simulink model "P3_Ex12b"  (R2018a)
settings: Solver=FixedStepAuto  StartTime=0.0  StopTime=30  RelTol=1e-3
PreLoadFcn:
  | % Plant
  | K0=0.82/0.017;
  | tau0=0.26;
  | N=9;
  | Kpot=1.62;
  | % Sampling period
  | Ts=0.01;
  | 
  | % Desired control specifications
  | Sp=80; % overshoot
  | Fd=0.5; % frequency
  | 
  | % Poles of the second order continuous system that will fulfill the specifications
  | wd=2*pi*Fd ;
  | xi=sqrt((log(Sp/100))^2/(pi^2+log(Sp/100)^2))
  | wn=wd/ sqrt(1-xi^2)
  | s1=-xi*wn+j*wd
  | s2=-xi*wn-j*wd
  | 
  | % Poles of the second order discrete system that will fulfill the specifications
  | p1=exp(Ts* s1 )
  | p2=exp(Ts* s2 )
  | % Fix third pole
  | p3=0.01
  | 
  | % Plant's Z transfere function
  | Ptas=tf([K0*(1/N)*Kpot],[tau0,1,0]);
  | Ptaz=c2d(Ptas,Ts,'zoh');
  | 
  | % Denominator and numerator coefficients
  | [Nz ,Dz]= tfdata(Ptaz,'v')
  | a1=Nz(2);
  | a0=Nz(3);
  | b1=Dz(2);
  | b0=Dz(3);
  | 
  | % A and B matrix definitions
  | A=[-1 -a1 -a1 -a1 ; p2+p3+p1 a1-a0 -a1-a0 -a0+2*a1 ; ...
  |    -p1*p2-p3*p1-p2*p3 a0 -a0 2*a0-a1 ; p1*p2*p3 0 0 -a0 ] ;
  | b=[p1+p2+p3-1+b1 ; -p1*p2-p3*p1-p3*p2+b0-b1 ; p1*p2*p3-b0 ; 0 ] ;
  | 
  | % x vector's determination of the controller
  | x=inv(A)*b ;
  | 
  | p4=x(1)
  | Kp=x(2)
  | Ki=(2/Ts)*x(3)
  | Kd=Ts*x(4)
  | pawd=0.2;
  | Kaw=1/Ki;
  | 
  | % Poles dominance calculation
  | dominancia=log(abs(p4))/log(abs(p1))
undefined symbols (not defined in the file or in its folder): DiscIntNeverNeededParam
libraries: arduinolib x2, simulink x2
settings Model: SimulationMode=external  ExtModeTrigDuration=2  Creator=Eneko Lerma  LastModifiedBy=Eneko Lerma
settings OptimizationCC: EnhancedBackFolding=on  PassReuseOutputArgsAs=Individual arguments  MaxStackSize=64  OptimizeBlockOrder=speed  DifferentSizesBufferReuse=on  OptimizationCustomize=off
settings DebuggingCC: ParameterPrecisionLossMsg=none  ParameterTunabilityLossMsg=error
settings HardwareCC: ProdBitPerPointer=32  ProdBitPerSizeT=32  ProdBitPerPtrDiffT=32  ProdLargestAtomicInteger=Long  ProdLargestAtomicFloat=Double  ProdWordSize=32  ProdHWDeviceType=ARM Compatible->ARM Cortex
settings SFSimCC: MATLABDynamicMemAlloc=off
settings RTWCC: SystemTargetFile=ert.tlc  HardwareBoard=Arduino Due  TLCOptions=-aInlineSetEventsForThisBaseRateFcn=TLC_FALSE -aSuppressMultiTaskScheduler=TLC_FALSE -aRateBasedStepFcn=1  TemplateMakefile=ert_default_tmf  GenerateReport=on  Toolchain=Arduino ARM  BuildConfiguration=Faster Runs  IncludeHyperlinkInReport=on  LaunchReport=on  GenerateTraceInfo=on  GenerateTraceReport=on  GenerateTraceReportSl=on  GenerateTraceReportSf=on  GenerateTraceReportEml=on
settings CodeAppCC: ForceParamTrailComments=on  IgnoreCustomStorageClasses=off  OperatorAnnotations=on  SimulinkDataObjDesc=on  SFDataObjDesc=on  InsertBlockDesc=on
settings ERTTargetCC: SupportContinuousTime=on  SupportVariableSizeSignals=on

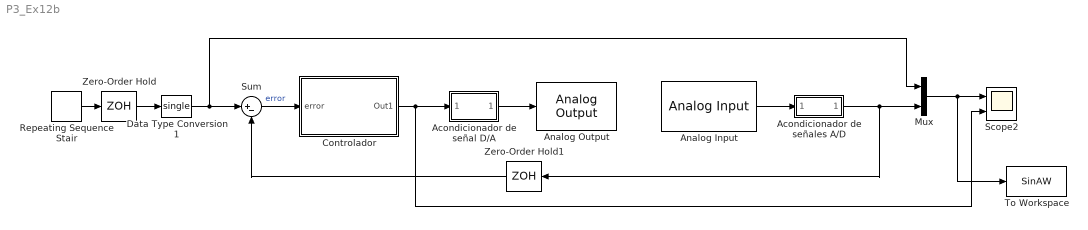
== system P3_Ex12b ==
  Acondicionador de señal D/A : Subsystem
  Acondicionador de señales A/D : Subsystem
  Analog Input : arduinolib/Analog Input  pinNumber=2  ReadResultsOnly=off  ConversionTriggerSource=Software  ExternalTriggerType=uint32(0)  OutputDataType=uint16  EnableConversionCompleteNotify=off  EnableOuputStatus=off  SampleTime=0.005  blockPlatform=arduino
  Analog Output : arduinolib/Analog Output  DACpin=DAC1  blockPlatform=arduino
      settings: SourceProductName=Simulink Support Package for Arduino Hardware  SourceProductBaseCode=ARDUINO
  Controlador : Subsystem
  Data Type Conversion1 : DataTypeConversion  OutDataTypeStr=single
  Mux : Mux  Inputs=2
  Repeating Sequence Stair : simulink/Sources/Repeating Sequence Stair  OutValues=[0 2 -2 -1].'  tsamp=4  OutMin=[]  OutMax=[]  OutDataTypeStr=double  OutputDataTypeScalingMode=double  OutDataType=fixdt(0,8)  ConRadixGroup=Best Precision: Vector-wise  OutScaling=2^-12
  Scope2 : Scope  NumInputPorts=2
  Sum : Sum  Inputs=|+-  AccumDataTypeStr=single
  To Workspace : ToWorkspace  VariableName=SinAW  SaveFormat=Structure With Time  SampleTime=-1
  Zero-Order Hold : ZeroOrderHold  SampleTime=Ts
  Zero-Order Hold1 : ZeroOrderHold  SampleTime=Ts
  wires:
  Mux/1 -> To Workspace/1, Scope2/1
  Repeating Sequence Stair/1 -> Zero-Order Hold/1
  Acondicionador de señales A/D/1(" ") -> Zero-Order Hold1/1, Mux/2
  Data Type Conversion1/1 -> Sum/1, Mux/1
  Sum/1 -> Controlador/1(error)  "error"
  Acondicionador de señal D/A/1(" ") -> Analog Output/1
  Analog Input/1 -> Acondicionador de señales A/D/1("  ")
  Controlador/1(Out1) -> Scope2/2, Acondicionador de señal D/A/1("  ")
  Zero-Order Hold/1 -> Data Type Conversion1/1
  Zero-Order Hold1/1 -> Sum/2

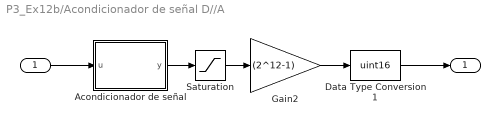
== system P3_Ex12b/Acondicionador de señal D//A ==
  "  " : Inport  OutDataTypeStr=double
  Acondicionador de señal : MATLAB Function  TreatAsAtomicUnit=on
  Data Type Conversion1 : DataTypeConversion  OutDataTypeStr=uint16
  Gain2 : Gain  Gain=(2^12-1)  OutDataTypeStr=single
  Saturation : Saturate  UpperLimit=1  LowerLimit=0  OutDataTypeStr=single
  " " : Outport  OutDataTypeStr=uint16
  wires:
  Gain2/1 -> Data Type Conversion1/1
  "  "/1 -> Acondicionador de señal/1(u)
  Acondicionador de señal/1(y) -> Saturation/1
  Data Type Conversion1/1 -> " "/1
  Saturation/1 -> Gain2/1

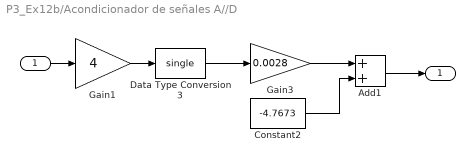
== system P3_Ex12b/Acondicionador de señales A//D ==
  "  " : Inport  OutDataTypeStr=uint16
  Add1 : Sum  AccumDataTypeStr=single
  Constant2 : Constant  Value=-4.7673  OutDataTypeStr=single
  Data Type Conversion3 : DataTypeConversion  OutDataTypeStr=single
  Gain1 : Gain  Gain=4  OutDataTypeStr=uint16
  Gain3 : Gain  Gain=0.0028  OutDataTypeStr=single
  " " : Outport  OutDataTypeStr=single
  wires:
  Gain1/1 -> Data Type Conversion3/1
  "  "/1 -> Gain1/1
  Data Type Conversion3/1 -> Gain3/1
  Gain3/1 -> Add1/1
  Constant2/1 -> Add1/2
  Add1/1 -> " "/1

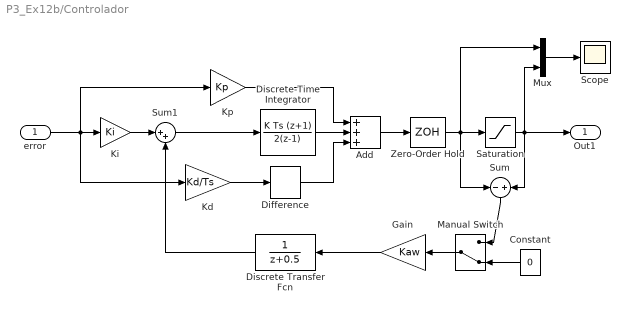
== system P3_Ex12b/Controlador ==
  error : Inport
  Add : Sum  Inputs=+++  AccumDataTypeStr=single
  Constant : Constant  Value=0  SampleTime=Ts
  Difference : simulink/Discrete/Difference  ICPrevInput=0.0  OutMin=[]  OutMax=[]  OutDataType=fixdt(1, 16)  OutScaling=2^-10  DoSatur=off
  Discrete Transfer Fcn : DiscreteTransferFcn  SampleTime=Ts
  Discrete-Time Integrator : DiscreteIntegrator  IntegratorMethod=Integration: Trapezoidal  SampleTime=Ts  ICPrevOutput=DiscIntNeverNeededParam  ICPrevScaledInput=DiscIntNeverNeededParam
  Gain : Gain  Gain=Kaw
  Kd : Gain  Gain=Kd/Ts
  Ki : Gain  Gain=Ki
  Kp : Gain  Gain=Kp
  Manual Switch : ManualSwitch  CurrentSetting=0
  Mux : Mux  Inputs=2
  Saturation : Saturate  UpperLimit=5  LowerLimit=-5  OutDataTypeStr=double
  Scope : Scope
  Sum : Sum  Inputs=-|+
  Sum1 : Sum  Inputs=|++
  Zero-Order Hold : ZeroOrderHold  SampleTime=Ts
  Out1 : Outport  OutDataTypeStr=double
  wires:
  Difference/1 -> Add/3
  Add/1 -> Zero-Order Hold/1
  Kp/1 -> Add/1
  Discrete-Time Integrator/1 -> Add/2
  Kd/1 -> Difference/1
  Sum1/1 -> Discrete-Time Integrator/1
  Sum/1 -> Manual Switch/1
  Manual Switch/1 -> Gain/1
  Constant/1 -> Manual Switch/2
  Zero-Order Hold/1 -> Mux/1, Sum/1, Saturation/1
  Gain/1 -> Discrete Transfer Fcn/1
  Discrete Transfer Fcn/1 -> Sum1/2
  Mux/1 -> Scope/1
  Saturation/1 -> Out1/1, Mux/2, Sum/2
  Ki/1 -> Sum1/1
  error/1 -> Ki/1, Kp/1, Kd/1

== matlab function P3_Ex12b/Acondicionador de señal D//A/Acondicionador de señal ==
  data: u input; y output
function y = fcn(u)
y =0.1342*u+0.3926;
